simulink model "prueba_flujocarga2_10_dic"  (R2015a)
settings: Solver=ode45  StartTime=0.0  StopTime=0.32  RelTol=1e-3
libraries: powerlib x34
settings Model: Creator=USUARIO  LastModifiedBy=USUARIO

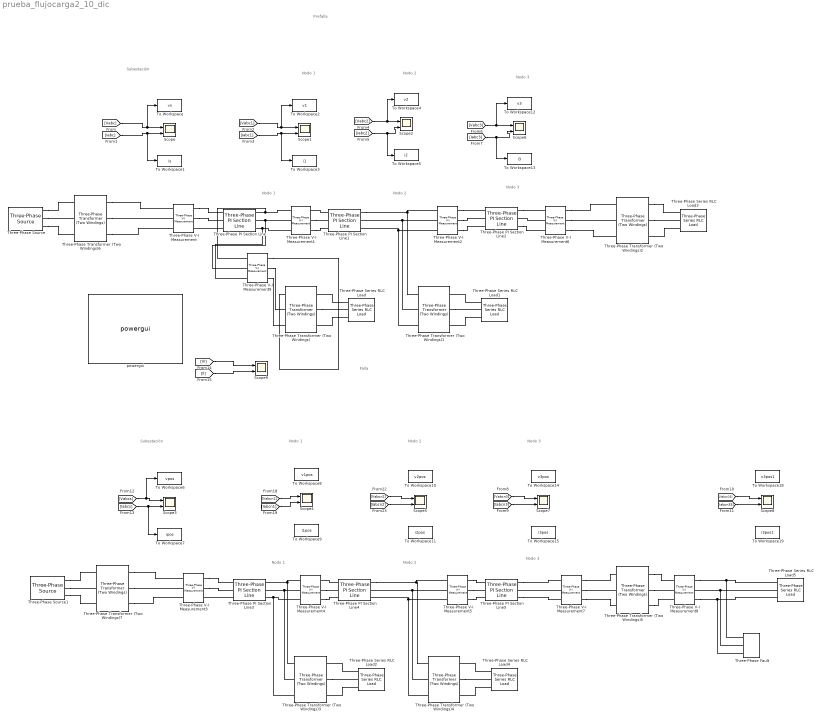
== system prueba_flujocarga2_10_dic ==
  note: Falla
  note: Prefalla
  note: Nodo 1
  note: Nodo 1
  note: Nodo 2
  note: Subestación
  note: Nodo 2
  note: Nodo 1
  note: Nodo 1
  note: Nodo 2
  note: Subestación
  note: Nodo 2
  note: Nodo 3
  note: Nodo 3
  note: Nodo 3
  note: Nodo 3
  Scope{,1..9} (10 alike) : Scope  NumInputPorts=2
      Scope settings: TickLabels=on  YMin=-120000~-175  YMax=120000~175
      Scope1 settings: TickLabels=on  YMin=-5~-5  YMax=5~5
      Scope2 settings: TickLabels=on  YMin=-5~-5  YMax=5~5  SaveName=ScopeData2
      Scope3 settings: TickLabels=on  TimeRange=0.008286453129078095  YMin=103212.4484142688~-4  YMax=109317.9377013964~5  SaveName=ScopeData3
      Scope4 settings: TickLabels=on  YMin=-5~-5  YMax=5~5  SaveName=ScopeData4
      Scope5 settings: TickLabels=on  YMin=-5~-5  YMax=5~5  SaveName=ScopeData5
      Scope6 settings: TickLabels=on  YMin=-5~-5  YMax=5~5  SaveName=ScopeData6
      Scope7 settings: TickLabels=on  YMin=-5~-5  YMax=5~5  SaveName=ScopeData7
      Scope8 settings: TickLabels=on  YMin=-5~-5  YMax=5~5  SaveName=ScopeData8
      Scope9 settings: TickLabels=on  YMin=-5~-5  YMax=5~5  SaveName=ScopeData9
  Three-Phase PI Section Line : powerlib/Elements/Three-Phase PI Section Line  LConnTagsString=a|b|c  RConnTagsString=A|B|C  Frequency=60  Resistances=[ 0.01273 0.3864]  Inductances="[ 0.9337e-3  4.1264e-3]"  Capacitances=[12.74e-9 7.751e-9]  Length=2
  Three-Phase PI Section Line1 : powerlib/Elements/Three-Phase PI Section Line  LConnTagsString=a|b|c  RConnTagsString=A|B|C  Frequency=60  Resistances=[ 0.01273 0.3864]  Inductances="[ 0.9337e-3  4.1264e-3]"  Capacitances=[12.74e-9 7.751e-9]  Length=1
  Three-Phase PI Section Line2 : powerlib/Elements/Three-Phase PI Section Line  LConnTagsString=a|b|c  RConnTagsString=A|B|C  Frequency=60  Resistances=[ 0.01273 0.3864]  Inductances="[ 0.9337e-3  4.1264e-3]"  Capacitances=[12.74e-9 7.751e-9]  Length=1.5
  Three-Phase PI Section Line3 : powerlib/Elements/Three-Phase PI Section Line  LConnTagsString=a|b|c  RConnTagsString=A|B|C  Frequency=60  Resistances=[ 0.01273 0.3864]  Inductances="[ 0.9337e-3  4.1264e-3]"  Capacitances=[12.74e-9 7.751e-9]  Length=2
  Three-Phase PI Section Line4 : powerlib/Elements/Three-Phase PI Section Line  LConnTagsString=a|b|c  RConnTagsString=A|B|C  Frequency=60  Resistances=[ 0.01273 0.3864]  Inductances="[ 0.9337e-3  4.1264e-3]"  Capacitances=[12.74e-9 7.751e-9]  Length=1
  Three-Phase PI Section Line5 : powerlib/Elements/Three-Phase PI Section Line  LConnTagsString=a|b|c  RConnTagsString=A|B|C  Frequency=60  Resistances=[ 0.01273 0.3864]  Inductances="[ 0.9337e-3  4.1264e-3]"  Capacitances=[12.74e-9 7.751e-9]  Length=1.5
  Three-Phase Series RLC Load{,1..5} (6 alike) : powerlib/Elements/Three-Phase Series RLC Load  LConnTagsString=A|B|C  Configuration=Y (grounded)  NominalVoltage=13800  NominalFrequency=60  ActivePower=75e3  InductivePower=100  CapacitivePower=100  Measurements=None  LoadType=constant Z
  Three-Phase Transformer (Two Windings){,1..3,5} (5 alike) : powerlib/Elements/Three-Phase Transformer (Two Windings)  Winding1Connection=Yg  Winding2Connection=Yg  CoreType=Three single-phase transformers  SetSaturation=off  Hysteresis=off  DataFile='hysteresis'  SetInitialFlux=off  Measurements=None  UNITS=pu  NominalPower=[ 75e3 , 60 ]  Winding1=[ 115e3 , 0.002 , 0.08 ]  Winding2=[ 13.8e3 , 0.002 , 0.08 ]  Rm=500  Lm=500  L0=0.5  Saturation=[ 0,0 ; 0.0024,1.2 ; 1.0,1.52 ]  InitialFluxes=[ 0.8 , -0.8 , 0.7 ]  MoreParameters=off  BreakLoop=off  DataType=off  TransfoNumber=1
  Three-Phase Transformer (Two Windings)4 : powerlib/Elements/Three-Phase Transformer (Two Windings)  Winding1Connection=Yg  Winding2Connection=Yg  CoreType=Three single-phase transformers  SetSaturation=off  Hysteresis=off  DataFile='hysteresis'  SetInitialFlux=off  Measurements=None  UNITS=pu  NominalPower=[ 75e3, 60 ]  Winding1=[ 115e3 , 0.002 , 0.08 ]  Winding2=[ 13.8e3 , 0.002 , 0.08 ]  Rm=500  Lm=500  L0=0.5  Saturation=[ 0,0 ; 0.0024,1.2 ; 1.0,1.52 ]  InitialFluxes=[ 0.8 , -0.8 , 0.7 ]  MoreParameters=off  BreakLoop=off  DataType=off  TransfoNumber=1
  Three-Phase Transformer (Two Windings)6 : powerlib/Elements/Three-Phase Transformer (Two Windings)  Winding1Connection=Yg  Winding2Connection=Yg  CoreType=Three single-phase transformers  SetSaturation=off  Hysteresis=off  DataFile='hysteresis'  SetInitialFlux=off  Measurements=None  UNITS=pu  NominalPower=[270e3 , 60 ]  Winding1=[ 13.8e3 , 0.002 , 0.08 ]  Winding2=[ 115e3, 0.002 , 0.08 ]  Rm=500  Lm=500  L0=0.5  Saturation=[ 0,0 ; 0.0024,1.2 ; 1.0,1.52 ]  InitialFluxes=[ 0.8 , -0.8 , 0.7 ]  MoreParameters=off  BreakLoop=off  DataType=off  TransfoNumber=1
  Three-Phase Transformer (Two Windings)7 : powerlib/Elements/Three-Phase Transformer (Two Windings)  Winding1Connection=Yg  Winding2Connection=Yg  CoreType=Three single-phase transformers  SetSaturation=off  Hysteresis=off  DataFile='hysteresis'  SetInitialFlux=off  Measurements=None  UNITS=pu  NominalPower=[270e3 , 60 ]  Winding1=[13800 0.002 0.080001]  Winding2=[1.15e+05 0.002 0.079999]  Rm=500  Lm=500  L0=0.5  Saturation=[0 0;0.0024 1.2;0.99999 1.52]  InitialFluxes=[0.80001 -0.80001 0.7]  MoreParameters=off  BreakLoop=off  DataType=off  TransfoNumber=1
  Three-Phase V-I Measurement : powerlib/Measurements/Three-Phase V-I Measurement  VoltageMeasurement=phase-to-ground  SetLabelV=on  LabelV=Vabc  Vpu=off  VpuLL=off  CurrentMeasurement=yes  SetLabelI=on  LabelI=Iabc  Ipu=off  Pbase=100e6  Vbase=500e3  OutputType=Complex  PhasorSimulation=off  PSBequivalent=0
  Three-Phase V-I Measurement1 : powerlib/Measurements/Three-Phase V-I Measurement  VoltageMeasurement=phase-to-ground  SetLabelV=on  LabelV=Vabc1  Vpu=off  VpuLL=off  CurrentMeasurement=yes  SetLabelI=on  LabelI=Iabc1  Ipu=off  Pbase=100e6  Vbase=500e3  OutputType=Complex  PhasorSimulation=off  PSBequivalent=0
  Three-Phase V-I Measurement2 : powerlib/Measurements/Three-Phase V-I Measurement  VoltageMeasurement=phase-to-ground  SetLabelV=on  LabelV=Vabc2  Vpu=off  VpuLL=off  CurrentMeasurement=yes  SetLabelI=on  LabelI=Iabc2  Ipu=off  Pbase=100e6  Vbase=500e3  OutputType=Complex  PhasorSimulation=off  PSBequivalent=0
  Three-Phase V-I Measurement3 : powerlib/Measurements/Three-Phase V-I Measurement  VoltageMeasurement=phase-to-ground  SetLabelV=on  LabelV=Vabcs  Vpu=off  VpuLL=off  CurrentMeasurement=yes  SetLabelI=on  LabelI=Iabcs  Ipu=off  Pbase=100e6  Vbase=500e3  OutputType=Complex  PhasorSimulation=off  PSBequivalent=0
  Three-Phase V-I Measurement4 : powerlib/Measurements/Three-Phase V-I Measurement  VoltageMeasurement=phase-to-ground  SetLabelV=on  LabelV=Vabcn1  Vpu=off  VpuLL=off  CurrentMeasurement=yes  SetLabelI=on  LabelI=Iabcn1  Ipu=off  Pbase=100e6  Vbase=500e3  OutputType=Complex  PhasorSimulation=off  PSBequivalent=0
  Three-Phase V-I Measurement5 : powerlib/Measurements/Three-Phase V-I Measurement  VoltageMeasurement=phase-to-ground  SetLabelV=on  LabelV=Vabcn2  Vpu=off  VpuLL=off  CurrentMeasurement=yes  SetLabelI=on  LabelI=Iabcn2  Ipu=off  Pbase=100e6  Vbase=500e3  OutputType=Complex  PhasorSimulation=off  PSBequivalent=0
  Three-Phase V-I Measurement6 : powerlib/Measurements/Three-Phase V-I Measurement  VoltageMeasurement=phase-to-ground  SetLabelV=on  LabelV=Vabc3  Vpu=off  VpuLL=off  CurrentMeasurement=yes  SetLabelI=on  LabelI=Iabc3  Ipu=off  Pbase=100e6  Vbase=500e3  OutputType=Complex  PhasorSimulation=off  PSBequivalent=0
  Three-Phase V-I Measurement7 : powerlib/Measurements/Three-Phase V-I Measurement  VoltageMeasurement=phase-to-ground  SetLabelV=on  LabelV=Vabcn3  Vpu=off  VpuLL=off  CurrentMeasurement=yes  SetLabelI=on  LabelI=Iabcn3  Ipu=off  Pbase=100e6  Vbase=500e3  OutputType=Complex  PhasorSimulation=off  PSBequivalent=0
  Three-Phase V-I Measurement8 : powerlib/Measurements/Three-Phase V-I Measurement  VoltageMeasurement=phase-to-ground  SetLabelV=on  LabelV=Vabcn33  Vpu=off  VpuLL=off  CurrentMeasurement=yes  SetLabelI=on  LabelI=Iabcn33  Ipu=off  Pbase=100e6  Vbase=500e3  OutputType=Complex  PhasorSimulation=off  PSBequivalent=0
  Three-Phase V-I Measurement9 : powerlib/Measurements/Three-Phase V-I Measurement  VoltageMeasurement=phase-to-ground  SetLabelV=on  LabelV=Vl  Vpu=off  VpuLL=off  CurrentMeasurement=yes  SetLabelI=on  LabelI=Il  Ipu=off  Pbase=100e6  Vbase=500e3  OutputType=Complex  PhasorSimulation=off  PSBequivalent=0
  Three-Phase Fault : powerlib/Elements/Three-Phase Fault  InitialStates=0  FaultA=on  FaultB=off  FaultC=off  GroundFault=on  SwitchTimes="[0.05  0.30]"  External=off  SwitchStatus=NaN  FaultResistance=0.01  GroundResistance=0.01  SnubberResistance=1e6  SnubberCapacitance=inf  Measurements=Fault currents
  Three-Phase Source : powerlib/Electrical Sources/Three-Phase Source  Voltage=13.8e3  PhaseAngle=0  Frequency=60  InternalConnection=Yg  SpecifyImpedance=on  Resistance=0.8929  Inductance=16.58e-3  ShortCircuitLevel=270e3  BaseVoltage=13.8  XRratio=7  BusType=swing  Pref=0  Qref=0  Qmin=-inf  Qmax=inf
  Three-Phase Source1 : powerlib/Electrical Sources/Three-Phase Source  Voltage=13.8e3  PhaseAngle=0  Frequency=60  InternalConnection=Yg  SpecifyImpedance=on  Resistance=0.8929  Inductance=16.58e-3  ShortCircuitLevel=100e6  BaseVoltage=13.8  XRratio=7  BusType=swing  Pref=0  Qref=0  Qmin=-inf  Qmax=inf
  To Workspace : ToWorkspace  VariableName=vs  SampleTime=-1
  To Workspace1 : ToWorkspace  VariableName=is  SampleTime=-1
  To Workspace10 : ToWorkspace  VariableName=v2pos  SampleTime=-1
  To Workspace11 : ToWorkspace  VariableName=i2pos  SampleTime=-1
  To Workspace12 : ToWorkspace  VariableName=v3  SampleTime=-1
  To Workspace13 : ToWorkspace  VariableName=i3  SampleTime=-1
  To Workspace14 : ToWorkspace  VariableName=v3pos  SampleTime=-1
  To Workspace15 : ToWorkspace  VariableName=i3pos  SampleTime=-1
  To Workspace18 : ToWorkspace  VariableName=v3pos1  SampleTime=-1
  To Workspace19 : ToWorkspace  VariableName=i3pos1  SampleTime=-1
  To Workspace2 : ToWorkspace  VariableName=v1  SampleTime=-1
  To Workspace3 : ToWorkspace  VariableName=i1  SampleTime=-1
  To Workspace4 : ToWorkspace  VariableName=v2  SampleTime=-1
  To Workspace5 : ToWorkspace  VariableName=i2  SampleTime=-1
  To Workspace6 : ToWorkspace  VariableName=vpos  SampleTime=-1
  To Workspace7 : ToWorkspace  VariableName=ipos  SampleTime=-1
  To Workspace8 : ToWorkspace  VariableName=v1pos  SampleTime=-1
  To Workspace9 : ToWorkspace  VariableName=i1pos  SampleTime=-1
  powergui : powerlib/powergui  Priority=1  SimulationMode=Discrete  SolverType=Tustin  SampleTime=5.208333e-4  frequency=60  SPID=off  DisableSnubberDevices=off  DisableRonSwitches=off  DisableVfSwitches=off  SwTol=0  DisplayEquations=off  Interpol=off  methode=off  Ts=0  FunctionMessages=off  echomessages=off  HookPort=off  EnableUseOfTLC=off  x0status=blocks  frequencyindice=60  Pbase=100e6  ErrMax=1e-4  Iterations=50  UnitsV=kV  UnitsW=MW  buscounter=0  RestoreLinks=warning  ResistiveCurrentMeasurement=off  Frange=[0:2:500]  Ylog=off  Xlog=on  ShowGrid=off  save=off  variable=ZData  structure=0  ZoomFFT=off  StartTime=0.0  cycles=1  DisplayStyle=1  fundamental=60  FreqAxis=off  MaxFrequency=1000  frequencyindicesteady=1  RmsSteady=1  display=off
  wires:
  [Vabc] -> To Workspace/1, Scope/1
  [Iabc] -> To Workspace1/1, Scope/2
  [Vabc1] -> To Workspace2/1, Scope1/1
  [Iabc1] -> To Workspace3/1, Scope1/2
  [Vabc2] -> To Workspace4/1, Scope2/1
  [Iabc2] -> To Workspace5/1, Scope2/2
  [Vabcs] -> To Workspace6/1, Scope3/1
  [Iabcs] -> To Workspace7/1, Scope3/2
  [Vabcn1] -> Scope4/1
  [Iabcn1] -> Scope4/2
  [Vabcn2] -> Scope5/1
  [Iabcn2] -> Scope5/2
  [Vabc3] -> To Workspace12/1, Scope6/1
  [Iabc3] -> To Workspace13/1, Scope6/2
  [Vabcn3] -> Scope7/1
  [Iabcn3] -> Scope7/2
  [Vabcn33] -> Scope8/1
  [Iabcn33] -> Scope8/2
  [Vl] -> Scope9/1
  [Il] -> Scope9/2
  connections:
  Three-Phase V-I Measurement1/LConn1 -- Three-Phase V-I Measurement9/LConn1 -- Three-Phase PI Section Line/RConn1
  Three-Phase V-I Measurement1/LConn2 -- Three-Phase V-I Measurement9/LConn2 -- Three-Phase PI Section Line/RConn2
  Three-Phase V-I Measurement1/LConn3 -- Three-Phase V-I Measurement9/LConn3 -- Three-Phase PI Section Line/RConn3
  Three-Phase PI Section Line1/RConn1 -- Three-Phase V-I Measurement2/LConn1 -- Three-Phase Transformer (Two Windings)1/LConn1
  Three-Phase Transformer (Two Windings)1/LConn2 -- Three-Phase V-I Measurement2/LConn2 -- Three-Phase PI Section Line1/RConn2
  Three-Phase Transformer (Two Windings)1/LConn3 -- Three-Phase V-I Measurement2/LConn3 -- Three-Phase PI Section Line1/RConn3
  Three-Phase V-I Measurement4/LConn1 -- Three-Phase Transformer (Two Windings)3/LConn1 -- Three-Phase PI Section Line3/RConn1
  Three-Phase V-I Measurement4/LConn2 -- Three-Phase Transformer (Two Windings)3/LConn2 -- Three-Phase PI Section Line3/RConn2
  Three-Phase V-I Measurement4/LConn3 -- Three-Phase Transformer (Two Windings)3/LConn3 -- Three-Phase PI Section Line3/RConn3
  Three-Phase PI Section Line4/RConn1 -- Three-Phase V-I Measurement5/LConn1 -- Three-Phase Transformer (Two Windings)4/LConn1
  Three-Phase Transformer (Two Windings)4/LConn2 -- Three-Phase V-I Measurement5/LConn2 -- Three-Phase PI Section Line4/RConn2
  Three-Phase Transformer (Two Windings)4/LConn3 -- Three-Phase V-I Measurement5/LConn3 -- Three-Phase PI Section Line4/RConn3
  Three-Phase Series RLC Load1/LConn3 -- Three-Phase Transformer (Two Windings)1/RConn3
  Three-Phase V-I Measurement/RConn1 -- Three-Phase PI Section Line/LConn1
  Three-Phase V-I Measurement/RConn2 -- Three-Phase PI Section Line/LConn2
  Three-Phase V-I Measurement2/RConn3 -- Three-Phase PI Section Line2/LConn3
  Three-Phase Series RLC Load/LConn1 -- Three-Phase Transformer (Two Windings)/RConn1
  Three-Phase V-I Measurement2/RConn2 -- Three-Phase PI Section Line2/LConn2
  Three-Phase PI Section Line1/LConn1 -- Three-Phase V-I Measurement1/RConn1
  Three-Phase V-I Measurement2/RConn1 -- Three-Phase PI Section Line2/LConn1
  Three-Phase V-I Measurement1/RConn2 -- Three-Phase PI Section Line1/LConn2
  Three-Phase Transformer (Two Windings)2/RConn1 -- Three-Phase Series RLC Load3/LConn1
  Three-Phase V-I Measurement1/RConn3 -- Three-Phase PI Section Line1/LConn3
  Three-Phase Transformer (Two Windings)1/RConn2 -- Three-Phase Series RLC Load1/LConn2
  Three-Phase Series RLC Load2/LConn3 -- Three-Phase Transformer (Two Windings)3/RConn3
  Three-Phase Series RLC Load4/LConn3 -- Three-Phase Transformer (Two Windings)4/RConn3
  Three-Phase PI Section Line3/LConn3 -- Three-Phase V-I Measurement3/RConn3
  Three-Phase Transformer (Two Windings)3/RConn2 -- Three-Phase Series RLC Load2/LConn2
  Three-Phase Transformer (Two Windings)2/RConn2 -- Three-Phase Series RLC Load3/LConn2
  Three-Phase Series RLC Load3/LConn3 -- Three-Phase Transformer (Two Windings)2/RConn3
  Three-Phase Series RLC Load1/LConn1 -- Three-Phase Transformer (Two Windings)1/RConn1
  Three-Phase Transformer (Two Windings)/RConn2 -- Three-Phase Series RLC Load/LConn2
  Three-Phase V-I Measurement5/RConn2 -- Three-Phase PI Section Line5/LConn2
  Three-Phase V-I Measurement5/RConn1 -- Three-Phase PI Section Line5/LConn1
  Three-Phase V-I Measurement5/RConn3 -- Three-Phase PI Section Line5/LConn3
  Three-Phase V-I Measurement4/RConn3 -- Three-Phase PI Section Line4/LConn3
  Three-Phase PI Section Line4/LConn1 -- Three-Phase V-I Measurement4/RConn1
  Three-Phase V-I Measurement4/RConn2 -- Three-Phase PI Section Line4/LConn2
  Three-Phase Transformer (Two Windings)4/RConn2 -- Three-Phase Series RLC Load4/LConn2
  Three-Phase Series RLC Load4/LConn1 -- Three-Phase Transformer (Two Windings)4/RConn1
  Three-Phase Series RLC Load2/LConn1 -- Three-Phase Transformer (Two Windings)3/RConn1
  Three-Phase V-I Measurement3/RConn2 -- Three-Phase PI Section Line3/LConn2
  Three-Phase V-I Measurement3/RConn1 -- Three-Phase PI Section Line3/LConn1
  Three-Phase Series RLC Load/LConn3 -- Three-Phase Transformer (Two Windings)/RConn3
  Three-Phase PI Section Line/LConn3 -- Three-Phase V-I Measurement/RConn3
  Three-Phase PI Section Line2/RConn1 -- Three-Phase V-I Measurement6/LConn1
  Three-Phase V-I Measurement6/LConn2 -- Three-Phase PI Section Line2/RConn2
  Three-Phase PI Section Line2/RConn3 -- Three-Phase V-I Measurement6/LConn3
  Three-Phase V-I Measurement6/RConn2 -- Three-Phase Transformer (Two Windings)2/LConn2
  Three-Phase V-I Measurement6/RConn1 -- Three-Phase Transformer (Two Windings)2/LConn1
  Three-Phase V-I Measurement6/RConn3 -- Three-Phase Transformer (Two Windings)2/LConn3
  Three-Phase PI Section Line5/RConn1 -- Three-Phase V-I Measurement7/LConn1
  Three-Phase V-I Measurement7/LConn2 -- Three-Phase PI Section Line5/RConn2
  Three-Phase PI Section Line5/RConn3 -- Three-Phase V-I Measurement7/LConn3
  Three-Phase V-I Measurement7/RConn2 -- Three-Phase Transformer (Two Windings)5/LConn2
  Three-Phase V-I Measurement7/RConn1 -- Three-Phase Transformer (Two Windings)5/LConn1
  Three-Phase V-I Measurement7/RConn3 -- Three-Phase Transformer (Two Windings)5/LConn3
  Three-Phase Transformer (Two Windings)5/RConn2 -- Three-Phase V-I Measurement8/LConn2
  Three-Phase Transformer (Two Windings)5/RConn3 -- Three-Phase V-I Measurement8/LConn3
  Three-Phase Transformer (Two Windings)5/RConn1 -- Three-Phase V-I Measurement8/LConn1
  Three-Phase V-I Measurement8/RConn1 -- Three-Phase Fault/LConn1 -- Three-Phase Series RLC Load5/LConn1
  Three-Phase Series RLC Load5/LConn2 -- Three-Phase Fault/LConn2 -- Three-Phase V-I Measurement8/RConn2
  Three-Phase V-I Measurement8/RConn3 -- Three-Phase Fault/LConn3 -- Three-Phase Series RLC Load5/LConn3
  Three-Phase V-I Measurement9/RConn1 -- Three-Phase Transformer (Two Windings)/LConn1
  Three-Phase V-I Measurement9/RConn2 -- Three-Phase Transformer (Two Windings)/LConn2
  Three-Phase V-I Measurement9/RConn3 -- Three-Phase Transformer (Two Windings)/LConn3
  Three-Phase Source/RConn2 -- Three-Phase Transformer (Two Windings)6/LConn2
  Three-Phase Source/RConn1 -- Three-Phase Transformer (Two Windings)6/LConn1
  Three-Phase Source/RConn3 -- Three-Phase Transformer (Two Windings)6/LConn3
  Three-Phase Transformer (Two Windings)6/RConn2 -- Three-Phase V-I Measurement/LConn2
  Three-Phase Transformer (Two Windings)6/RConn1 -- Three-Phase V-I Measurement/LConn1
  Three-Phase Transformer (Two Windings)6/RConn3 -- Three-Phase V-I Measurement/LConn3
  Three-Phase Source1/RConn3 -- Three-Phase Transformer (Two Windings)7/LConn3
  Three-Phase Source1/RConn1 -- Three-Phase Transformer (Two Windings)7/LConn1
  Three-Phase Source1/RConn2 -- Three-Phase Transformer (Two Windings)7/LConn2
  Three-Phase Transformer (Two Windings)7/RConn2 -- Three-Phase V-I Measurement3/LConn2
  Three-Phase Transformer (Two Windings)7/RConn3 -- Three-Phase V-I Measurement3/LConn3
  Three-Phase Transformer (Two Windings)7/RConn1 -- Three-Phase V-I Measurement3/LConn1
